simulink model "DR18E_Testpult"  (R2017a)
settings: Solver=ode1  StartTime=0.0  StopTime=Inf  FixedStep=0.001  RelTol=1e-3
PostLoadFcn:
  | , if any(exist('dsrtsu_mdlpostloadfcn', 'file') == [2, 3, 6]), try dsrtsu_mdlpostloadfcn('Execute', bdroot); catch fprintf('Error in PostLoadFcn (dsrtsu_mdlpostloadfcn) for model "%s":\n %s\n', bdroot, lasterr); end, end,
model workspace: external: MAT-File C:\Users\DeltaRacing\Documents\dSPACE\MABX_DR18E\Model\DR18E_MABX_Parameter.mat (data not in the file)
values from neighbouring files (symbols this model uses):
  am = 1/Ts    (= 1)    [DR18E_MABX_Parameter.m]
  bm = K/Ts    (= 0.05)    [DR18E_MABX_Parameter.m]
  cf = 41350    [DR18E_MABX_Parameter.m]
  cr = 41350    [DR18E_MABX_Parameter.m]
  Derating_HV_Battery_Kapa = 1    [DR18E_MABX_Parameter.m]
  Derating_Start_km = 16    [DR18E_MABX_Parameter.m]
  Drive_Mode = 0    [DR18E_MABX_Parameter.m]
  g = 1    [DR18E_MABX_Parameter.m]
  Gas_Modus = 2    [DR18E_MABX_Parameter.m]
  HV_Power_max = 80    [DR18E_MABX_Parameter.m]
  i_Getriebe = 3.3    [DR18E_MABX_Parameter.m]
  i_Lenkgetriebe = 4.32    [DR18E_MABX_Parameter.m]
  K_SET = 1    [DR18E_MABX_Parameter.m]
  Kapazitaet_HV_Battery_kWh = 6.6    [DR18E_MABX_Parameter.m]
  KW_T_Soll = 37    [DR18E_MABX_Parameter.m]
  lf = 1.2    [DR18E_MABX_Parameter.m]
  lr = 1.15    [DR18E_MABX_Parameter.m]
  m = mdriver + mvehicle    (= 310)    [DR18E_MABX_Parameter.m]
  M_max = 150    [DR18E_MABX_Parameter.m]
  Power_Limit_onoff = 0    [DR18E_MABX_Parameter.m]
  Reifenradius = 0.2351    [DR18E_MABX_Parameter.m]
  Strecke_Endu_km = 22    [DR18E_MABX_Parameter.m]
  TC_Decr_Gas = 0.00005    (= 5e-05)    [DR18E_MABX_Parameter.m]
  TC_Derivative = 0.4    [DR18E_MABX_Parameter.m]
  TC_Incr_Gas = 0.005    [DR18E_MABX_Parameter.m]
  TC_On = 0    [DR18E_MABX_Parameter.m]
  TC_Relay_Off = 0.065    [DR18E_MABX_Parameter.m]
  TC_Relay_On = 0.07    [DR18E_MABX_Parameter.m]
  TV_Mode = 2    [DR18E_MABX_Parameter.m]
  TV_On = 0    [DR18E_MABX_Parameter.m]
  TV_Override = 1    [DR18E_MABX_Parameter.m]
  y = 0.8    [DR18E_MABX_Parameter.m]
undefined symbols (not defined in the file or in its folder): D, DiscIntNeverNeededParam, I, K_OL, P
libraries: simulink x288, rtican x100, rtiusbflightreclib x40, rti1401lib_dio_type3 x10, simulink_extras x10, rti1401lib_adc_type4 x8, rti1401lib_II_base x7
(part 14 of 27)

== system DR18E_Testpult/Eingabe Fahrzeug/BMS/Voltage 9-10 ==
  Timeout : Inport
  Bus Creator : BusCreator  Inputs=2
  Logical Operator : Logic  Operator=OR  AllPortsSameDT=off  OutDataTypeStr=boolean
  Voltage Stack 10 : Subsystem
  Voltage Stack 9 : Subsystem
  Cell97-120 : Outport
  TimeoutError : Outport  Port=2
  wires:
  Timeout/1 -> Voltage Stack 10/1(Timeout[samples]), Voltage Stack 9/1(Timeout[samples])
  Voltage Stack 10/2(TimeoutError) -> Logical Operator/2
  Bus Creator/1 -> Cell97-120/1  "Cell97-120"
  Voltage Stack 10/1(Cell97-108) -> Bus Creator/2  "Cell109-120"
  Voltage Stack 9/1(Cell97-108) -> Bus Creator/1  "Cell97-108"
  Voltage Stack 9/2(TimeoutError) -> Logical Operator/1
  Logical Operator/1 -> TimeoutError/1

== system DR18E_Testpult/Eingabe Fahrzeug/BMS/Voltage Stack 1-2 ==
  Timeout : Inport
  Bus Creator : BusCreator  Inputs=2
  Logical Operator : Logic  Operator=OR  AllPortsSameDT=off  OutDataTypeStr=boolean
  Voltage Stack 1 : Subsystem
  Voltage Stack 2 : Subsystem
  Cell1-24 : Outport
  TimeoutError : Outport  Port=2
  wires:
  Timeout/1 -> Voltage Stack 2/1(Timeout[samples]), Voltage Stack 1/1(Timeout[samples])
  Voltage Stack 2/2(TimeoutError) -> Logical Operator/2
  Bus Creator/1 -> Cell1-24/1  "Cell1-24"
  Voltage Stack 2/1(Cell1-12) -> Bus Creator/2  "Cell13-24"
  Voltage Stack 1/1(Cell1-12) -> Bus Creator/1  "Cell1-12"
  Voltage Stack 1/2(TimeoutError) -> Logical Operator/1
  Logical Operator/1 -> TimeoutError/1

== system DR18E_Testpult/Eingabe Fahrzeug/BMS/Voltage Stack 3-4 ==
  Timeout : Inport
  Bus Creator : BusCreator  Inputs=2
  Logical Operator : Logic  Operator=OR  AllPortsSameDT=off  OutDataTypeStr=boolean
  Voltage Stack 3 : Subsystem
  Voltage Stack 4 : Subsystem
  Cell25-48 : Outport
  TimeoutError : Outport  Port=2
  wires:
  Timeout/1 -> Voltage Stack 4/1(Timeout[samples]), Voltage Stack 3/1(Timeout[samples])
  Voltage Stack 4/2(TimeoutError) -> Logical Operator/2
  Bus Creator/1 -> Cell25-48/1  "Cell25-48"
  Voltage Stack 4/1(Cell37-48) -> Bus Creator/2  "Cell37-48"
  Voltage Stack 3/1(Cell25-36) -> Bus Creator/1  "Cell25-36"
  Voltage Stack 3/2(TimeoutError) -> Logical Operator/1
  Logical Operator/1 -> TimeoutError/1

== system DR18E_Testpult/Eingabe Fahrzeug/BMS/Voltage Stack 5-6 ==
  Timeout : Inport
  Bus Creator : BusCreator  Inputs=2
  Logical Operator : Logic  Operator=OR  AllPortsSameDT=off  OutDataTypeStr=boolean
  Voltage Stack 5 : Subsystem
  Voltage Stack 6 : Subsystem
  Cell49-72 : Outport
  TimeoutError : Outport  Port=2
  wires:
  Timeout/1 -> Voltage Stack 6/1(Timeout[samples]), Voltage Stack 5/1(Timeout[samples])
  Voltage Stack 6/2(TimeoutError) -> Logical Operator/2
  Bus Creator/1 -> Cell49-72/1  "Cell49-72"
  Voltage Stack 6/1(Cell49-60) -> Bus Creator/2  "Cell61-72"
  Voltage Stack 5/1(Cell49-60) -> Bus Creator/1  "Cell49-60"
  Voltage Stack 5/2(TimeoutError) -> Logical Operator/1
  Logical Operator/1 -> TimeoutError/1

== system DR18E_Testpult/Eingabe Fahrzeug/BMS/Voltage Stack 7-8 ==
  Timeout : Inport
  Bus Creator : BusCreator  Inputs=2
  Logical Operator : Logic  Operator=OR  AllPortsSameDT=off  OutDataTypeStr=boolean
  Voltage Stack 7 : Subsystem
  Voltage Stack 8 : Subsystem
  "Cell73-96 " : Outport
  TimeoutError : Outport  Port=2
  wires:
  Timeout/1 -> Voltage Stack 8/1(Timeout[samples]), Voltage Stack 7/1(Timeout[samples])
  Voltage Stack 8/2(TimeoutError) -> Logical Operator/2
  Bus Creator/1 -> "Cell73-96 "/1  "Cell73-96"
  Voltage Stack 8/1(Cell73-84) -> Bus Creator/2  "Cell85-96"
  Voltage Stack 7/1(Cell73-84) -> Bus Creator/1  "Cell73-84"
  Voltage Stack 7/2(TimeoutError) -> Logical Operator/1
  Logical Operator/1 -> TimeoutError/1

== system DR18E_Testpult/Eingabe Fahrzeug/CAN IO/RX OK Detection1 ==
  note: This subsystem surveys if the sending of the TX message is successful and if it meets the
      | requirements concerning the regularity of the sending.
      |
      | If for 5 consecutive execution steps the message could not be successfully sent the 'TX Warn'
      | output is set to 1. Also, the message is expected to be sent every 50 ms approximatively. If this
      | condition is not met 5 times consecutively the 'TX Warn' output is set to 1.
  TX status : Inport
  TX delta time : Inport  Port=2
  Delta time limit : Constant  Value=0.055
  Delta time limit exceeded : RelationalOperator  RndMeth=Nearest  InputSameDT=on
  Mem{1..4} (4 alike) : Memory
  OR : Logic  Operator=OR
  Prev. msg. not sent : RelationalOperator  Operator=~=  RndMeth=Nearest  InputSameDT=on
  Prev. msg. sent value : Constant
  Warn : Logic  Inputs=5
  TX Warn : Outport
  wires:
  TX delta time/1 -> Delta time limit exceeded/1
  Delta time limit/1 -> Delta time limit exceeded/2
  Prev. msg. sent value/1 -> Prev. msg. not sent/2
  TX status/1 -> Prev. msg. not sent/1
  Prev. msg. not sent/1 -> OR/1
  Delta time limit exceeded/1 -> OR/2
  OR/1 -> Mem1/1, Warn/1
  Mem1/1 -> Mem2/1, Warn/2
  Mem2/1 -> Mem3/1, Warn/3
  Mem3/1 -> Mem4/1, Warn/4
  Mem4/1 -> Warn/5
  Warn/1 -> TX Warn/1

== system DR18E_Testpult/Eingabe Fahrzeug/CAN IO/RX OK Detection3 ==
  note: This subsystem surveys if the sending of the TX message is successful and if it meets the
      | requirements concerning the regularity of the sending.
      |
      | If for 5 consecutive execution steps the message could not be successfully sent the 'TX Warn'
      | output is set to 1. Also, the message is expected to be sent every 50 ms approximatively. If this
      | condition is not met 5 times consecutively the 'TX Warn' output is set to 1.
  TX status : Inport
  TX delta time : Inport  Port=2
  Delta time limit : Constant  Value=0.055
  Delta time limit exceeded : RelationalOperator  RndMeth=Nearest  InputSameDT=on
  Mem{1..4} (4 alike) : Memory
  OR : Logic  Operator=OR
  Prev. msg. not sent : RelationalOperator  Operator=~=  RndMeth=Nearest  InputSameDT=on
  Prev. msg. sent value : Constant
  Warn : Logic  Inputs=5
  TX Warn : Outport
  wires:
  TX delta time/1 -> Delta time limit exceeded/1
  Delta time limit/1 -> Delta time limit exceeded/2
  Prev. msg. sent value/1 -> Prev. msg. not sent/2
  TX status/1 -> Prev. msg. not sent/1
  Prev. msg. not sent/1 -> OR/1
  Delta time limit exceeded/1 -> OR/2
  OR/1 -> Mem1/1, Warn/1
  Mem1/1 -> Mem2/1, Warn/2
  Mem2/1 -> Mem3/1, Warn/3
  Mem3/1 -> Mem4/1, Warn/4
  Mem4/1 -> Warn/5
  Warn/1 -> TX Warn/1

== system DR18E_Testpult/Eingabe Fahrzeug/Gyro/FlightRecorder4 ==
  In1 : Inport
  Data Type Conversion : DataTypeConversion
  Gain : Gain
  USB_FLIGHT_REC_BL1 : rtiusbflightreclib/USB_FLIGHT_REC_BL1  VarName=Gierrate  DataType=Single  SampleTime=-1  TLCFileName=rtiusbflightrecwrite  Reserved1=[]  Reserved2=[]  Reserved3=[]  Reserved4=[]  DSProperties=struct('RTI',struct('Version',uint32(3),'BlockType',struct('isSLSource',uint8(0),'isSLSink',uint8(1),'isHWSource',uint8(0),'isHWSink',uint8(0),'isSetup',uint8(0),'isInline',uint8(1),'isNonInline',uint8(0),'isInterrupt',uint8(0),'isChannelwise',uint8(0)),'IOBoardType',{{'DSUSB','FLIGHTREC'}},'UnitType','FLIGHTREC','Identifier','WRITE','DialogType','SL','BlockSet','RTIUSBFLIGHTREC','SlaveProcessor','NONE'))  RTIBlockInterface=struct('InputPortsActive',1,'InputPortsWidth',int32(1),'InputPortsDataType',{{'SS_SINGLE'}},'BlockDisplay',{{['Write to\nUSB Flight Recorder'],'center'}},'IconTransparency','off','InitLevel',3,'BlockName',struct('Token',{{'USB_FLIGHT_REC_BL1'}}),'MaskDescription',['Write input to the Flight Recorder. Recorded data can be referenced by the specified variable.'],'SampleTime',{{-1}})  RTIBlockParameters=struct('VarName',{{'Gierrate','OFF',[]}},'DataType',{{'Single','OFF',[]}},'SampleTime',{{-1,'OFF',[]}},'TLCFileName',{{'rtiusbflightrecwrite','OFF',[]}})  RTISFcnParameters=struct('VarName','char','DataType','char','SampleTime','double','TLCFileName','char')  RTIBlockParaDefault=struct('VarName','Var1','DataType','Single','SampleTime',-1,'TLCFileName','rtiusbflightrecwrite')
      settings: SourceProductName=dSPACE RTI USB Flight Rec Blockset
  wires:
  Data Type Conversion/1 -> USB_FLIGHT_REC_BL1/1
  In1/1 -> Gain/1
  Gain/1 -> Data Type Conversion/1

== system DR18E_Testpult/Eingabe Fahrzeug/Gyro/RX Timeout Detection ==
  RX status : Inport
  Timeout (n Samples) : Inport  Port=2
  Terminator_4 : Terminator
  Triggered Subsystem : Subsystem  TreatAsAtomicUnit=on
  RX Timeout Error : Outport
  wires:
  RX status/1 -> Triggered Subsystem/1(TXStatus)
  Triggered Subsystem/1(Rampe) -> Terminator_4/1
  Triggered Subsystem/2(RX Timeout Error) -> RX Timeout Error/1  "RX Timeout"
  Timeout (n Samples)/1 -> Triggered Subsystem/2(Timeout)

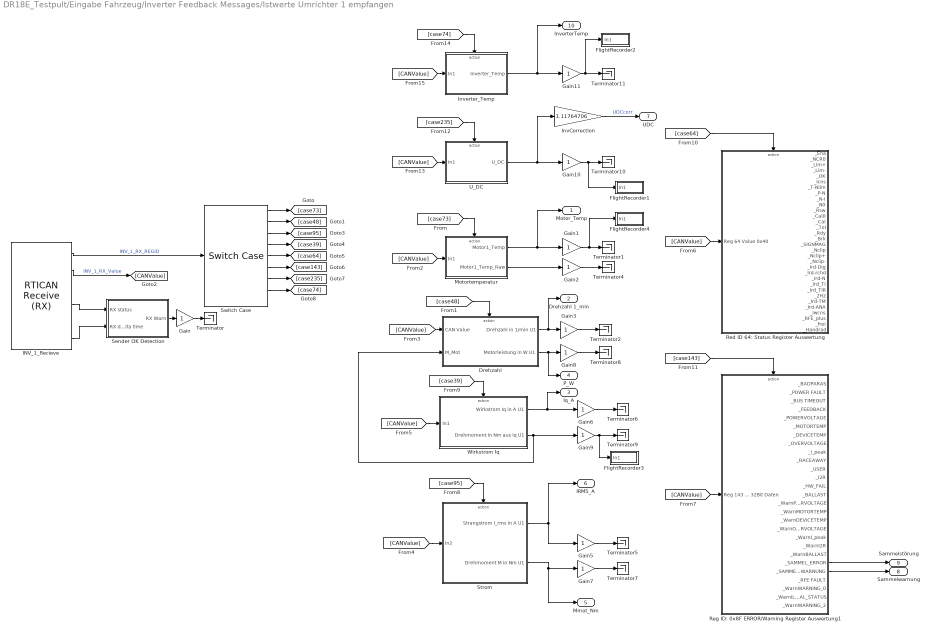
== system DR18E_Testpult/Eingabe Fahrzeug/Inverter Feedback Messages/Istwerte Umrichter 1 empfangen  ==
  Drehzahl : Subsystem  TreatAsAtomicUnit=on
  FlightRecorder1 : Subsystem
  FlightRecorder2 : Subsystem
  FlightRecorder3 : Subsystem
  FlightRecorder4 : Subsystem
  Gain{,1..3,5..11} (11 alike) : Gain
  INV_1_Recieve : rtican/RTICAN Receive (RX)   Reserved1=[]  Reserved2=[]  Reserved3=[]  Reserved4=[]  SfcnMessage=[]  Msg_Struct=[]  BoardTypeNo=[]  BoardNo=[]  ChannelNo=[]  Parameters=[]  DialogFcn=[]  UnitName=[]  Revision=[]  UnitValues=[]  DSProperties=struct('RTI',struct('Version',uint32(5),'BlockType',struct('isSLSource',uint8(1),'isSLSink',uint8(1),'isHWSource',uint8(0),'isHWSink',uint8(0),'isSetup',uint8(0),'isInline',uint8(1),'isNonInline',uint8(0),'isInterrupt',uint8(0),'isChannelwise',uint8(0)),'IOBoardType','RTICAN','UnitType','MESSAGE','Identifier','RX','DialogType','MSVC','BlockSet','RTICAN','SlaveProcessor','CAN'))  RTIBlockInterface=struct('OutputPortsWidth',int32([1 1 1 1 1 1]),'OutputPortsActive',[1 1 1 1 1 1],'OutputPortsName',{{'INV_1_RX_REGID','INV_1_RX_Value','muell',['RX status'],['RX time'],['RX delta time']}},'OutputPortsDataType',{{'SS_DOUBLE','SS_DOUBLE','SS_DOUBLE','SS_DOUBLE','SS_DOUBLE','SS_DOUBLE'}},'OutputPortsLabel',{{'INV_1_RX_REGID','INV_1_RX_Value','muell','','',''}},'OutputPortsLabelMode','ON','InputPortsWidth',int32(0),'InputPortsActive',0,'DialogFcn','rtican_message_interface_gui','BlockDisplay',{{'','center'}},'IconTransparency','on','ParameterTunableNames',{{}},'InitLevel',3,'BlockName',struct('Token',{{'INV_1_Recieve'}}),'SampleTime',{{-1}},'TriggerPort',{{'none'}},'EnablePort',{{'none'}})  RTIBlockParameters=struct('BoardTypeNo',{{1,'OFF',[]}},'BoardNo',{{1,'ON',[1 16]}},'ChannelNo',{{1,'ON',[1 2]}},'Parameters',{{struct('DataFileSupport',struct('DataFileSelectedMaster',0,'DataFileSelectedLocal',0,'DataFileName',['<no datafile support>|'],'DataFileDate',['01-Aug-2018 13:44:51'],'SelectedFile',['<no file selected>'],'InterfaceFcn','rtican_dbc_file_parser'),'Options',struct('StatusSelected',1,'TimeSelected',1,'DeltaTimeSelected',1,'BytePortSelected',0,'MessageLengthSelected',0,'TriggerPort',struct('Selected',0,'TriggerType',0),'UserCoding',struct('Selected',0,'InterfaceFile','UserDecodingFile','FcnName','UserDecodeFcn','InportSelected',0,'InportWidth',1,'OutportSelected',0,'OutportWidth',1),'EnablePortSelected',0,'SignalOnPortnameSelected',1,'UseRXService',0),'Message',struct('MsgOnBlocknameSelected',1,'MsgName','INV_1_Recieve','MsgIdFormat',0,'MsgId',273,'MsgLength',6,'NumSignals',3,'SampleTime',-1,'Signal',struct('SgnName',{'INV_1_RX_REGID','INV_1_RX_Value','muell'},'SgnStartBit',{0,8,40},'SgnLength',{8,16,8},'SgnType',{0,0,0},'ModeValue',{-1,-1,-1},'DataType',{0,0,0},'ByteLayout',{0,0,0},'Factor',{1,1,1},'Offset',{0,0,0},'SgnComment',{{''},{''},{''}},'SgnUnit',{'','',''},'Min',{0,0,0},'Max',{0,0,0},'SLDataType',{'SS_DOUBLE','SS_DOUBLE','SS_DOUBLE'}),'MsgIdNumFormat',1,'MsgComment',{{''}}),'Version',1.2,'general',struct('isFromLib',0)),'OFF',[]}},'GroupId',{{struct('Group',{{'RTICAN'}},'No',2,'Behavior',{{'NAMECHANGE'}},'BlockType',{{'SINK'}},'NameChangeFlag',0),'OFF',[]}},'SFcnRTICANMessage',{{struct('MsgType','RX','SFcnPortType','Scalar','MsgName','INV_1_Recieve','MsgIdFormat','STD','MsgId',273,'MsgLength',6,'NumSignals',3,'SampleTime',-1,'Signal',struct('SgnName',{'INV_1_RX_REGID','INV_1_RX_Value','muell'},'SgnStartBit',{0,8,40},'SgnLength',{8,16,8},'SgnType',{'standard','standard','standard'},'ModeValue',{-1,-1,-1},'DataType',{['unsigned int'],['unsigned int'],['unsigned int']},'ByteLayout',{['little endian'],['little endian'],['little endian']},'Factor',{1,1,1},'Offset',{0,0,0},'SLDataType',{'SS_DOUBLE','SS_DOUBLE','SS_DOUBLE'}),'StatusSelected','yes','TimeSelected','yes','DeltaTimeSelected','yes','BytePortSelected','no','MessageLengthSelected','no','TriggerPort',struct('Selected','no','TriggerType',0),'UserCoding',struct('Selected','no','InterfaceFile','UserDecodingFile','FcnName','UserDecodeFcn','InportSelected','no','InportWidth',1,'OutportSelected','no','OutportWidth',1),'EnablePortSelected','no','UseRXService','no','BoardType','DS1','BoardNo',1,'ControllerNo',1),'OFF',[]}},'TLCFileName',{{'rtican_rx_message','OFF',[]}})  RTISFcnParameters=struct('SFcnRTICANMessage','struct','TLCFileName','char')  RTIBlockParaDefault=struct('BoardTypeNo',4302,'BoardNo',1,'ChannelNo',1,'Parameters',struct('DataFileSupport',struct('DataFileSelectedMaster',0,'DataFileSelectedLocal',0,'DataFileName','','DataFileDate','','SelectedFile',['<no file selected>']),'Options',struct('StatusSelected',1,'TimeSelected',1,'DeltaTimeSelected',1,'BytePortSelected',0,'MessageLengthSelected',0,'TriggerPort',struct('Selected',0,'TriggerType','rising'),'UserCoding',struct('Selected',0,'InterfaceFile','UserDecodingFile','FcnName','UserDecodeFcn','InportSelected',0,'InportWidth',1,'OutportSelected',0,'OutportWidth',1),'EnablePortSelected',0,'SignalOnPortnameSelected',1,'UseRXService',0),'Message',struct('MsgOnBlocknameSelected',0,'MsgName',['RX Message'],'MsgIdFormat',0,'MsgId',100,'MsgLength',8,'NumSignals',1,'SampleTime',-1,'Signal',struct('SgnName',['RX signal'],'SgnStartBit',0,'SgnLength',8,'SgnType',0,'ModeValue',-1,'DataType',0,'SLDataType','SS_DOUBLE','ByteLayout',0,'Factor',1,'Offset',0,'Min',0,'Max',255,'SgnComment',{{}},'SgnUnit',''),'MsgIdNumFormat',0,'MsgComment',{{''}}),'Version',1.2,'general',struct('isFromLib',1)),'GroupId',struct('Group',{{'RTICAN'}},'No',1,'Behavior',{{'NAMECHANGE'}},'BlockType',{{'SINK'}},'NameChangeFlag',0),'SFcnRTICANMessage',struct('MsgType','RX','MsgName',['RX Message'],'MsgIdFormat','STD','MsgId',100,'MsgLength',8,'NumSignals',1,'SampleTime',-1,'Signal',struct('SgnName',['RX signal'],'SgnStartBit',0,'SgnLength',8,'SgnType','standard','ModeValue',-1,'DataType',['unsigned int'],'ByteLayout',['little endian'],'SLDataType','SS_DOUBLE','Factor',1,'Offset',0),'StatusSelected','yes','TimeSelected','yes','DeltaTimeSelected','yes','BytePortSelected','no','MessageLengthSelected','no','EnablePortSelected','no','UserCoding',struct('Selected','no','InterfaceFile','UserDecodingFile','FcnName','UserDecodeFcn','InportSelected','no','InportWidth',1,'OutportSelected','no','OutportWidth',1),'TriggerPort',struct('Selected','no','TriggerType','rising'),'UseRXService','no','BoardType','DS4302','BoardNo',1,'ControllerNo',1,'SFcnPortType','Scalar'),'TLCFileName','rtican_rx_message')
      settings: AttributesFormatString=Group Id: RTICAN2\n  SourceProductName=dSPACE RTI CAN Blockset
  InvCorrection : Gain  Gain=1.11764706
  Inverter_Temp : Subsystem  TreatAsAtomicUnit=on
  Motortemperatur : Subsystem  TreatAsAtomicUnit=on
  Red ID 64: Status Register Auswertung : Subsystem  TreatAsAtomicUnit=on
  Reg ID: 0x8F ERROR/Warning Register Auswertung1 : Subsystem  TreatAsAtomicUnit=on
  Sender OK Detection : Subsystem
  Strom : Subsystem  TreatAsAtomicUnit=on
  Switch Case : SwitchCase  CaseConditions={hex2dec('0049'),hex2dec('0030'),hex2dec('005F'),hex2dec('27'),64,hex2dec('8F'),hex2dec('EB'),hex2dec('4A')}
  Terminator{,1..2,4..11} (11 alike) : Terminator
  U_DC : Subsystem  TreatAsAtomicUnit=on
  Wirkstrom Iq : Subsystem  TreatAsAtomicUnit=on
  Motor_Temp : Outport
  Drehzahl 1_min : Outport  Port=2
  Iq_A : Outport  Port=3
  P_W : Outport  Port=4
  Mmot_Nm : Outport  Port=5
  IRMS_A : Outport  Port=6
  UDC : Outport  Port=7
  Sammelwarnung : Outport  Port=8
  Sammelstörung : Outport  Port=9
  InverterTemp : Outport  Port=10
  wires:
  Gain1/1 -> FlightRecorder4/1(In1), Terminator1/1
  Motortemperatur/2("Motor1_Temp_Raw ") -> Gain2/1
  Gain2/1 -> Terminator4/1
  Gain3/1 -> Terminator2/1
  Gain5/1 -> Terminator5/1
  Gain6/1 -> Terminator6/1
  Wirkstrom Iq/1(Wirkstrom Iq in A U1) -> Iq_A/1, Gain6/1
  Strom/1(Strangstrom I_rms in A U1) -> Gain5/1, IRMS_A/1
  Gain7/1 -> Terminator7/1
  Strom/2(Drehmoment M in Nm U1) -> Mmot_Nm/1, Gain7/1
  Gain8/1 -> Terminator8/1
  Drehzahl/1(Drehzahl in 1/min U1) -> Drehzahl 1_min/1, Gain3/1
  Drehzahl/2(Motorleistung in W U1) -> P_W/1, Gain8/1
  Sender OK Detection/1(RX Warn) -> Gain/1
  Gain/1 -> Terminator/1
  INV_1_Recieve/4 -> Sender OK Detection/1(RX status)
  INV_1_Recieve/6 -> Sender OK Detection/2(RX delta time)
  Gain9/1 -> FlightRecorder3/1(In1), Terminator9/1
  Wirkstrom Iq/2(Drehmoment in Nm aus Iq U1) -> Drehzahl/2(M_Mot), Gain9/1
  Switch Case/1 -> [case73]
  [case73] -> Motortemperatur/Action
  Switch Case/2 -> [case48]
  [case48] -> Drehzahl/Action
  [CANValue] -> Motortemperatur/1(In1)
  [CANValue] -> Drehzahl/1(CAN Value)
  [CANValue] -> Strom/1(In2)
  [CANValue] -> Wirkstrom Iq/1(In1)
  [CANValue] -> Red ID 64: Status Register Auswertung/1(Reg 64 Value 0x40)
  [CANValue] -> Reg ID: 0x8F ERROR/Warning Register Auswertung1/1(Reg 143 Value 0x8F 32Bit Daten)
  Switch Case/3 -> [case95]
  [case95] -> Strom/Action
  Switch Case/4 -> [case39]
  [case39] -> Wirkstrom Iq/Action
  [case64] -> Red ID 64: Status Register Auswertung/Action
  Switch Case/5 -> [case64]
  Switch Case/6 -> [case143]
  [case143] -> Reg ID: 0x8F ERROR/Warning Register Auswertung1/Action
  Motortemperatur/1(Motor1_Temp) -> Motor_Temp/1, Gain1/1
  Reg ID: 0x8F ERROR/Warning Register Auswertung1/23(_SAMMEL_WARNUNG) -> Sammelwarnung/1
  Reg ID: 0x8F ERROR/Warning Register Auswertung1/22(_SAMMEL_ERROR) -> Sammelstörung/1
  Switch Case/7 -> [case235]
  Gain10/1 -> FlightRecorder1/1(In1), Terminator10/1
  [case235] -> U_DC/Action
  [CANValue] -> U_DC/1(In1)
  U_DC/1(U_DC) -> InvCorrection/1, Gain10/1
  Switch Case/8 -> [case74]
  Gain11/1 -> FlightRecorder2/1(In1), Terminator11/1
  [case74] -> Inverter_Temp/Action
  [CANValue] -> Inverter_Temp/1(In1)
  Inverter_Temp/1(Inverter_Temp) -> InverterTemp/1, Gain11/1
  InvCorrection/1 -> UDC/1  "UDCcorr"
  INV_1_Recieve/2 -> [CANValue]  "INV_1_RX_Value"
  INV_1_Recieve/1 -> Switch Case/1  "INV_1_RX_REGID"

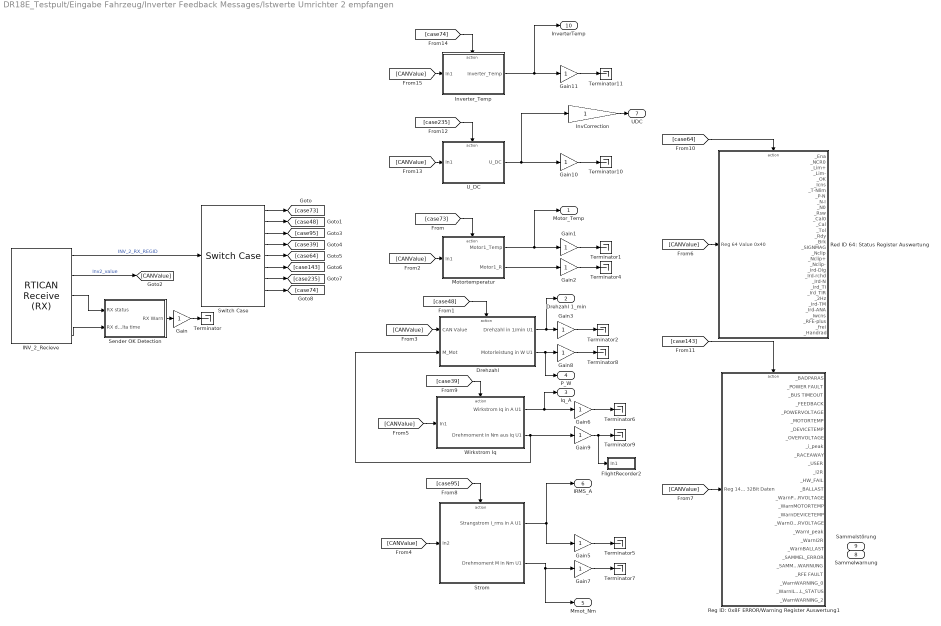
== system DR18E_Testpult/Eingabe Fahrzeug/Inverter Feedback Messages/Istwerte Umrichter 2 empfangen ==
  Drehzahl : Subsystem  TreatAsAtomicUnit=on
  FlightRecorder2 : Subsystem
  Gain{,1..3,5..11} (11 alike) : Gain
  INV_2_Recieve : rtican/RTICAN Receive (RX)   Reserved1=[]  Reserved2=[]  Reserved3=[]  Reserved4=[]  SfcnMessage=[]  Msg_Struct=[]  BoardTypeNo=[]  BoardNo=[]  ChannelNo=[]  Parameters=[]  DialogFcn=[]  UnitName=[]  Revision=[]  UnitValues=[]  DSProperties=struct('RTI',struct('Version',uint32(5),'BlockType',struct('isSLSource',uint8(1),'isSLSink',uint8(1),'isHWSource',uint8(0),'isHWSink',uint8(0),'isSetup',uint8(0),'isInline',uint8(1),'isNonInline',uint8(0),'isInterrupt',uint8(0),'isChannelwise',uint8(0)),'IOBoardType','RTICAN','UnitType','MESSAGE','Identifier','RX','DialogType','MSVC','BlockSet','RTICAN','SlaveProcessor','CAN'))  RTIBlockInterface=struct('OutputPortsWidth',int32([1 1 1 1 1]),'OutputPortsActive',[1 1 1 1 1],'OutputPortsName',{{'INV_2_RX_REGID','Inv2_value',['RX status'],['RX time'],['RX delta time']}},'OutputPortsDataType',{{'SS_DOUBLE','SS_DOUBLE','SS_DOUBLE','SS_DOUBLE','SS_DOUBLE'}},'OutputPortsLabel',{{'INV_2_RX_REGID','Inv2_value','','',''}},'OutputPortsLabelMode','ON','InputPortsWidth',int32(0),'InputPortsActive',0,'DialogFcn','rtican_message_interface_gui','BlockDisplay',{{'','center'}},'IconTransparency','on','ParameterTunableNames',{{}},'InitLevel',3,'BlockName',struct('Token',{{'INV_2_Recieve'}}),'SampleTime',{{-1}},'TriggerPort',{{'none'}},'EnablePort',{{'none'}})  RTIBlockParameters=struct('BoardTypeNo',{{1,'OFF',[]}},'BoardNo',{{1,'ON',[1 16]}},'ChannelNo',{{2,'ON',[1 2]}},'Parameters',{{struct('DataFileSupport',struct('DataFileSelectedMaster',0,'DataFileSelectedLocal',0,'DataFileName',['<no datafile support>|'],'DataFileDate',['01-Aug-2018 13:44:51'],'SelectedFile',['<no file selected>'],'InterfaceFcn','rtican_dbc_file_parser'),'Options',struct('StatusSelected',1,'TimeSelected',1,'DeltaTimeSelected',1,'BytePortSelected',0,'MessageLengthSelected',0,'TriggerPort',struct('Selected',0,'TriggerType',0),'UserCoding',struct('Selected',0,'InterfaceFile','UserDecodingFile','FcnName','UserDecodeFcn','InportSelected',0,'InportWidth',1,'OutportSelected',0,'OutportWidth',1),'EnablePortSelected',0,'SignalOnPortnameSelected',1,'UseRXService',0),'Message',struct('MsgOnBlocknameSelected',1,'MsgName','INV_2_Recieve','MsgIdFormat',0,'MsgId',274,'MsgLength',6,'NumSignals',2,'SampleTime',-1,'Signal',struct('SgnName',{'INV_2_RX_REGID','Inv2_value'},'SgnStartBit',{0,8},'SgnLength',{8,16},'SgnType',{0,0},'ModeValue',{-1,-1},'DataType',{0,0},'ByteLayout',{0,0},'Factor',{1,1},'Offset',{0,0},'SgnComment',{{''},{''}},'SgnUnit',{'',''},'Min',{0,0},'Max',{0,0},'SLDataType',{'SS_DOUBLE','SS_DOUBLE'}),'MsgIdNumFormat',1,'MsgComment',{{''}}),'Version',1.2,'general',struct('isFromLib',0)),'OFF',[]}},'GroupId',{{struct('Group',{{'RTICAN'}},'No',3,'Behavior',{{'NAMECHANGE'}},'BlockType',{{'SINK'}},'NameChangeFlag',0),'OFF',[]}},'SFcnRTICANMessage',{{struct('MsgType','RX','SFcnPortType','Scalar','MsgName','INV_2_Recieve','MsgIdFormat','STD','MsgId',274,'MsgLength',6,'NumSignals',2,'SampleTime',-1,'Signal',struct('SgnName',{'INV_2_RX_REGID','Inv2_value'},'SgnStartBit',{0,8},'SgnLength',{8,16},'SgnType',{'standard','standard'},'ModeValue',{-1,-1},'DataType',{['unsigned int'],['unsigned int']},'ByteLayout',{['little endian'],['little endian']},'Factor',{1,1},'Offset',{0,0},'SLDataType',{'SS_DOUBLE','SS_DOUBLE'}),'StatusSelected','yes','TimeSelected','yes','DeltaTimeSelected','yes','BytePortSelected','no','MessageLengthSelected','no','TriggerPort',struct('Selected','no','TriggerType',0),'UserCoding',struct('Selected','no','InterfaceFile','UserDecodingFile','FcnName','UserDecodeFcn','InportSelected','no','InportWidth',1,'OutportSelected','no','OutportWidth',1),'EnablePortSelected','no','UseRXService','no','BoardType','DS1','BoardNo',1,'ControllerNo',2),'OFF',[]}},'TLCFileName',{{'rtican_rx_message','OFF',[]}})  RTISFcnParameters=struct('SFcnRTICANMessage','struct','TLCFileName','char')  RTIBlockParaDefault=struct('BoardTypeNo',4302,'BoardNo',1,'ChannelNo',1,'Parameters',struct('DataFileSupport',struct('DataFileSelectedMaster',0,'DataFileSelectedLocal',0,'DataFileName','','DataFileDate','','SelectedFile',['<no file selected>']),'Options',struct('StatusSelected',1,'TimeSelected',1,'DeltaTimeSelected',1,'BytePortSelected',0,'MessageLengthSelected',0,'TriggerPort',struct('Selected',0,'TriggerType','rising'),'UserCoding',struct('Selected',0,'InterfaceFile','UserDecodingFile','FcnName','UserDecodeFcn','InportSelected',0,'InportWidth',1,'OutportSelected',0,'OutportWidth',1),'EnablePortSelected',0,'SignalOnPortnameSelected',1,'UseRXService',0),'Message',struct('MsgOnBlocknameSelected',0,'MsgName',['RX Message'],'MsgIdFormat',0,'MsgId',100,'MsgLength',8,'NumSignals',1,'SampleTime',-1,'Signal',struct('SgnName',['RX signal'],'SgnStartBit',0,'SgnLength',8,'SgnType',0,'ModeValue',-1,'DataType',0,'SLDataType','SS_DOUBLE','ByteLayout',0,'Factor',1,'Offset',0,'Min',0,'Max',255,'SgnComment',{{}},'SgnUnit',''),'MsgIdNumFormat',0,'MsgComment',{{''}}),'Version',1.2,'general',struct('isFromLib',1)),'GroupId',struct('Group',{{'RTICAN'}},'No',1,'Behavior',{{'NAMECHANGE'}},'BlockType',{{'SINK'}},'NameChangeFlag',0),'SFcnRTICANMessage',struct('MsgType','RX','MsgName',['RX Message'],'MsgIdFormat','STD','MsgId',100,'MsgLength',8,'NumSignals',1,'SampleTime',-1,'Signal',struct('SgnName',['RX signal'],'SgnStartBit',0,'SgnLength',8,'SgnType','standard','ModeValue',-1,'DataType',['unsigned int'],'ByteLayout',['little endian'],'SLDataType','SS_DOUBLE','Factor',1,'Offset',0),'StatusSelected','yes','TimeSelected','yes','DeltaTimeSelected','yes','BytePortSelected','no','MessageLengthSelected','no','EnablePortSelected','no','UserCoding',struct('Selected','no','InterfaceFile','UserDecodingFile','FcnName','UserDecodeFcn','InportSelected','no','InportWidth',1,'OutportSelected','no','OutportWidth',1),'TriggerPort',struct('Selected','no','TriggerType','rising'),'UseRXService','no','BoardType','DS4302','BoardNo',1,'ControllerNo',1,'SFcnPortType','Scalar'),'TLCFileName','rtican_rx_message')
      settings: AttributesFormatString=Group Id: RTICAN3\n  SourceProductName=dSPACE RTI CAN Blockset
  InvCorrection : Gain
  Inverter_Temp : Subsystem  TreatAsAtomicUnit=on
  Motortemperatur : Subsystem  TreatAsAtomicUnit=on
  Red ID 64: Status Register Auswertung : Subsystem  TreatAsAtomicUnit=on
  Reg ID: 0x8F ERROR/Warning Register Auswertung1 : Subsystem  TreatAsAtomicUnit=on
  Sender OK Detection : Subsystem
  Strom : Subsystem  TreatAsAtomicUnit=on
  Switch Case : SwitchCase  CaseConditions={hex2dec('0049'),hex2dec('0030'),hex2dec('005F'),hex2dec('27'),64,hex2dec('8F'),hex2dec('EB'),hex2dec('4A')}
  Terminator{,1..2,4..11} (11 alike) : Terminator
  U_DC : Subsystem  TreatAsAtomicUnit=on
  Wirkstrom Iq : Subsystem  TreatAsAtomicUnit=on
  Motor_Temp : Outport
  Drehzahl 1_min : Outport  Port=2
  Iq_A : Outport  Port=3
  P_W : Outport  Port=4
  Mmot_Nm : Outport  Port=5
  IRMS_A : Outport  Port=6
  UDC : Outport  Port=7
  Sammelwarnung : Outport  Port=8
  Sammelstörung : Outport  Port=9
  InverterTemp : Outport  Port=10
  wires:
  Gain1/1 -> Terminator1/1
  Motortemperatur/2("Motor1_R ") -> Gain2/1
  Gain2/1 -> Terminator4/1
  Gain3/1 -> Terminator2/1
  Gain5/1 -> Terminator5/1
  Gain6/1 -> Terminator6/1
  Wirkstrom Iq/1(Wirkstrom Iq in A U1) -> Iq_A/1, Gain6/1
  Strom/1(Strangstrom I_rms in A U1) -> Gain5/1, IRMS_A/1
  Gain7/1 -> Terminator7/1
  Strom/2(Drehmoment M in Nm U1) -> Mmot_Nm/1, Gain7/1
  Gain8/1 -> Terminator8/1
  Drehzahl/1(Drehzahl in 1/min U1) -> Drehzahl 1_min/1, Gain3/1
  Drehzahl/2(Motorleistung in W U1) -> P_W/1, Gain8/1
  Sender OK Detection/1(RX Warn) -> Gain/1
  Gain/1 -> Terminator/1
  INV_2_Recieve/3 -> Sender OK Detection/1(RX status)
  INV_2_Recieve/5 -> Sender OK Detection/2(RX delta time)
  Gain9/1 -> FlightRecorder2/1(In1), Terminator9/1
  Wirkstrom Iq/2(Drehmoment in Nm aus Iq U1) -> Drehzahl/2(M_Mot), Gain9/1
  Switch Case/1 -> [case73]
  [case73] -> Motortemperatur/Action
  Switch Case/2 -> [case48]
  [case48] -> Drehzahl/Action
  [CANValue] -> Motortemperatur/1(In1)
  [CANValue] -> Drehzahl/1(CAN Value)
  [CANValue] -> Strom/1(In2)
  [CANValue] -> Wirkstrom Iq/1(In1)
  [CANValue] -> Red ID 64: Status Register Auswertung/1(Reg 64 Value 0x40)
  [CANValue] -> Reg ID: 0x8F ERROR/Warning Register Auswertung1/1(Reg 143 Value 0x8F 32Bit Daten)
  Switch Case/3 -> [case95]
  [case95] -> Strom/Action
  Switch Case/4 -> [case39]
  [case39] -> Wirkstrom Iq/Action
  [case64] -> Red ID 64: Status Register Auswertung/Action
  Switch Case/5 -> [case64]
  Switch Case/6 -> [case143]
  [case143] -> Reg ID: 0x8F ERROR/Warning Register Auswertung1/Action
  Motortemperatur/1(Motor1_Temp) -> Motor_Temp/1, Gain1/1
  ? -> Sammelwarnung/1
  ? -> Sammelstörung/1
  Switch Case/7 -> [case235]
  Gain10/1 -> Terminator10/1
  [case235] -> U_DC/Action
  [CANValue] -> U_DC/1(In1)
  U_DC/1(U_DC) -> InvCorrection/1, Gain10/1
  Switch Case/8 -> [case74]
  Gain11/1 -> Terminator11/1
  [case74] -> Inverter_Temp/Action
  [CANValue] -> Inverter_Temp/1(In1)
  Inverter_Temp/1(Inverter_Temp) -> InverterTemp/1, Gain11/1
  InvCorrection/1 -> UDC/1
  INV_2_Recieve/1 -> Switch Case/1  "INV_2_RX_REGID"
  INV_2_Recieve/2 -> [CANValue]  "Inv2_value"

== system DR18E_Testpult/Eingabe Fahrzeug/Lenkwinkelgeber/FlightRecorder ==
  In1 : Inport
  Data Type Conversion : DataTypeConversion
  Gain : Gain
  USB_FLIGHT_REC_BL1 : rtiusbflightreclib/USB_FLIGHT_REC_BL1  VarName=Lenkwinkel  DataType=Single  SampleTime=-1  TLCFileName=rtiusbflightrecwrite  Reserved1=[]  Reserved2=[]  Reserved3=[]  Reserved4=[]  DSProperties=struct('RTI',struct('Version',uint32(3),'BlockType',struct('isSLSource',uint8(0),'isSLSink',uint8(1),'isHWSource',uint8(0),'isHWSink',uint8(0),'isSetup',uint8(0),'isInline',uint8(1),'isNonInline',uint8(0),'isInterrupt',uint8(0),'isChannelwise',uint8(0)),'IOBoardType',{{'DSUSB','FLIGHTREC'}},'UnitType','FLIGHTREC','Identifier','WRITE','DialogType','SL','BlockSet','RTIUSBFLIGHTREC','SlaveProcessor','NONE'))  RTIBlockInterface=struct('InputPortsActive',1,'InputPortsWidth',int32(1),'InputPortsDataType',{{'SS_SINGLE'}},'BlockDisplay',{{['Write to\nUSB Flight Recorder'],'center'}},'IconTransparency','off','InitLevel',3,'BlockName',struct('Token',{{'USB_FLIGHT_REC_BL1'}}),'MaskDescription',['Write input to the Flight Recorder. Recorded data can be referenced by the specified variable.'],'SampleTime',{{-1}})  RTIBlockParameters=struct('VarName',{{'Lenkwinkel','OFF',[]}},'DataType',{{'Single','OFF',[]}},'SampleTime',{{-1,'OFF',[]}},'TLCFileName',{{'rtiusbflightrecwrite','OFF',[]}})  RTISFcnParameters=struct('VarName','char','DataType','char','SampleTime','double','TLCFileName','char')  RTIBlockParaDefault=struct('VarName','Var1','DataType','Single','SampleTime',-1,'TLCFileName','rtiusbflightrecwrite')
      settings: SourceProductName=dSPACE RTI USB Flight Rec Blockset
  wires:
  Data Type Conversion/1 -> USB_FLIGHT_REC_BL1/1
  In1/1 -> Gain/1
  Gain/1 -> Data Type Conversion/1

== system DR18E_Testpult/Eingabe Fahrzeug/Lenkwinkelgeber/RX Timeout Detection ==
  RX status : Inport
  Timeout (n Samples) : Inport  Port=2
  Terminator_4 : Terminator
  Triggered Subsystem : Subsystem  TreatAsAtomicUnit=on
  RX Timeout Error : Outport
  wires:
  RX status/1 -> Triggered Subsystem/1(TXStatus)
  Triggered Subsystem/1(Rampe) -> Terminator_4/1
  Triggered Subsystem/2(RX Timeout Error) -> RX Timeout Error/1  "RX Timeout"
  Timeout (n Samples)/1 -> Triggered Subsystem/2(Timeout)
